simulink model "part4"  (R2019a)
settings: Solver=VariableStepAuto  StartTime=0.0  StopTime=10.0  RelTol=1e-3
settings Model: Creator=G5  LastModifiedBy=G5

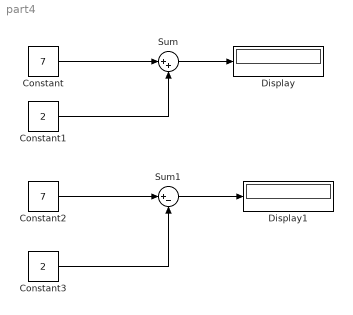
== system part4 ==
  Constant : Constant  Value=7
  Constant1 : Constant  Value=2
  Constant2 : Constant  Value=7
  Constant3 : Constant  Value=2
  Display : Display
  Display1 : Display
  Sum : Sum  Inputs=|++
  Sum1 : Sum  Inputs=|+-
  wires:
  Constant/1 -> Sum/1
  Constant1/1 -> Sum/2
  Sum/1 -> Display/1
  Sum1/1 -> Display1/1
  Constant3/1 -> Sum1/2
  Constant2/1 -> Sum1/1
